simulink model "commpcccvs"  (R2023b)
settings: Solver=FixedStepDiscrete  StartTime=0.0  StopTime=360  RelTol=1e-3
PostLoadFcn:
  | %Default parameters
  | prmPcccVs.blkLength1 = 1024;
  | prmPcccVs.blkLength2 = 4096;
  | prmPcccVs.EbNo = 0.7;
  | prmPcccVs.numIter = 6;
  | 
  | % Derived parameter
  | prmPcccVs.maxBlkLength = max(prmPcccVs.blkLength1, prmPcccVs.blkLength2);
undefined symbols (not defined in the file or in its folder): gCRC24B, getTurboIOIndices
libraries: commsink2 x2, commdigbbndpm3 x2, commcrc2 x2, commrandsrc3 x2, dspsrcs4 x2, commcnvcod2 x2, commchan3 x1
Description:
  | Variable-sized Turbo Coding
  | 
  | Companion to the commpccc model, this model highlights Turbo coding with variable-sized signals in Simulink.
  | Using the 3GPP TS 36.212 v9.0 specifications for the Turbo encoder and decoder, the example
  | highlights the performance variations with different code block lengths.
  | 
  | The model can be configured to run with any two of the 188 code block sizes supported by the standard
  | and is set to evaluate the code block error performance over an AWGN channel.
settings Model: FPTRunName=Active  Creator=The MathWorks, Inc.  LastModifiedBy=yuvra
settings SolverCC: AlgebraicLoopSolver=TrustRegion
settings DataIOCC: LimitDataPoints=on  SaveFormat=Array  SaveOutput=off  SignalLogging=off  DSMLogging=off  SaveTime=off  ReturnWorkspaceOutputs=off
settings OptimizationCC: ReuseModelBlockBuffer=off  ExpressionDepthLimit=2147483647  RollThreshold=2  LifeSpan=inf  SimCompilerOptimization=on
settings DebuggingCC: UnderspecifiedInitializationDetection=Classic  MergeDetectMultiDrivingBlocksExec=none  SolverPrmCheckMsg=warning  FcnCallInpInsideContextMsg=warning  UnconnectedInputMsg=warning  UnconnectedOutputMsg=warning  UnconnectedLineMsg=warning  AllowSymbolicDim=off  StateNameClashWarn=warning  SFUnexpectedBacktrackingDiag=warning  SFNoUnconditionalDefaultTransitionDiag=warning  SFExecutionAtInitializationDiag=none  ArithmeticOperatorsInVariantConditions=warning
settings HardwareCC: ProdBitPerPointer=32  ProdBitPerSizeT=32  ProdBitPerPtrDiffT=32  ProdLargestAtomicFloat=None  ProdIntDivRoundTo=Undefined  ProdEndianess=Unspecified  ProdWordSize=32  ProdHWDeviceType=32-bit Generic
settings ModelReferenceCC: EnableRefExpFcnMdlSchedulingChecks=on  PropagateSignalLabelsOutOfModel=off
settings SFSimCC: SFSimEcho=off  SimCtrlC=off  SimIntegrity=off  SimUseLocalCustomCode=off  CustomCodeUndefinedFunction=UseInterfaceOnly
settings RTWCC: RTWUseLocalCustomCode=off  DLArmComputeVersion=19.05
settings CodeAppCC: StateflowObjectComments=on
settings GRTTargetCC: TargetLangStandard=C89/C90 (ANSI)  CombineOutputUpdateFcns=off  GRTInterface=on
settings ConfigComp: CovMetricSettings=dw  CovSaveCumulativeToWorkspaceVar=on  CovSaveSingleToWorkspaceVar=on  CovExternalEMLEnable=off  CovSFcnEnable=off

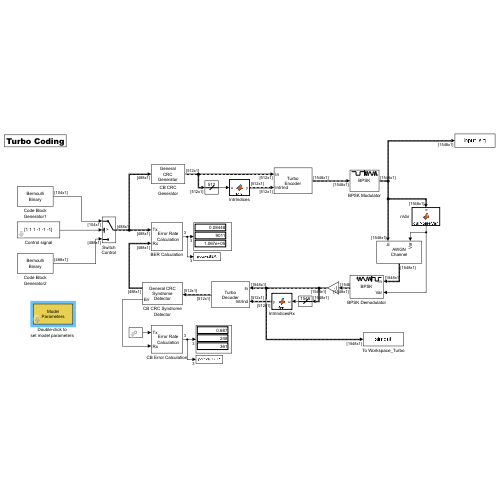
[thumbnail: Simulink's stored preview of the top-level diagram]
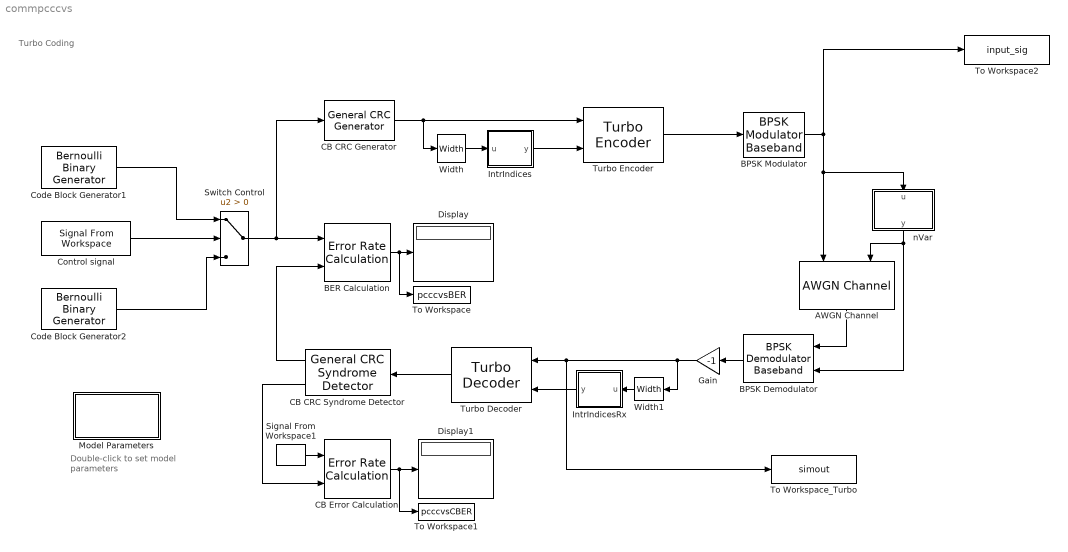
== system commpcccvs ==
  note: Turbo Coding
  note: Double-click to
      | set model parameters
  AWGN Channel : commchan3/AWGN Channel  LegacyMode=off  NoiseMethod=Variance  noiseMode=Variance from port  EbNo=10  EsNo=10  SNR=10  BitsPerSymbol=1  SignalPower=1  SamplesPerSymbol=1  SymbolPeriod=1  VarianceSource=Input port  Variance=1  RandomStream=mt19937ar with seed  Seed=98765  SimulateUsing=Code generation
  BER Calculation : commsink2/Error Rate Calculation  N=0  st_delay=0  cp_mode=Entire frame  subframe=[]  PMode=Port  WsName=ErrorVec1  RsMode2=off  stop=off  numErr=maxNumErrs  maxBits=maxNumBits
  BPSK Demodulator : commdigbbndpm3/BPSK Demodulator Baseband  DecType=Log-likelihood ratio  VarSource=Port  Variance=1  Ph=0  outDtype=Inherit via internal rule  derotateFactorWordLen=16  derotateFactorDataTypeStr=Inherit: Same word length as input  derotateFactorLastDataTypeStr=Inherit: Same word length as input
  BPSK Modulator : commdigbbndpm3/BPSK Modulator Baseband  Ph=0  outDtype=double  outWordLen=16  outUDDataType=sfix(16)  outFracLenMode=Best precision  outFracLen=15  outDataTypeStr=double  outLastDataTypeStr=double
  CB CRC Generator : commcrc2/General CRC Generator  genPoly=[1 1 zeros(1, 16) 1 1 0 0 0 1 1] % gCRC24B  iniStates=0  directMethod=off  reflectInputBytes=off  reflectChecksums=off  finalXOR=0  numChecksums=1
  CB CRC Syndrome Detector : commcrc2/General CRC Syndrome Detector  genPoly=[1 1 zeros(1, 16) 1 1 0 0 0 1 1] % gCRC24B  iniStates=0  directMethod=off  reflectInputBytes=off  reflectChecksums=off  finalXOR=0  numChecksums=1
  CB Error Calculation : commsink2/Error Rate Calculation  N=0  st_delay=0  cp_mode=Entire frame  subframe=[]  PMode=Port  WsName=ErrorVec1  RsMode2=off  stop=off  numErr=maxNumErrs  maxBits=maxNumBits
  Code Block Generator1 : commrandsrc3/Bernoulli Binary Generator  ProbabilityOfZero=0.5  SeedSource=Parameter  Seed=12345  SampleTime=1/(prmPcccVs.blkLength1-24)  SamplesPerFrame=prmPcccVs.blkLength1-24  OutputDataType=double  SimulateUsing=Interpreted execution
  Code Block Generator2 : commrandsrc3/Bernoulli Binary Generator  ProbabilityOfZero=0.5  SeedSource=Parameter  Seed=67890  SampleTime=1/(prmPcccVs.blkLength2-24)  SamplesPerFrame=prmPcccVs.blkLength2-24  OutputDataType=double  SimulateUsing=Interpreted execution
  Control signal : dspsrcs4/Signal From Workspace  X=[1 1 1 -1 -1 -1]  Ts=1  nsamps=1  OutputAfterFinalValue=Cyclic repetition  ignoreOrWarnInputAndFrameLengths=off  OutputFrames=on
  Display : Display
  Display1 : Display
  Gain : Gain  Gain=-1
  IntrIndices : MATLAB Function  TreatAsAtomicUnit=on
  IntrIndicesRx : MATLAB Function  TreatAsAtomicUnit=on
  Model Parameters : Subsystem  mask(Model Parameters){blkLength1=128, blkLength2=512, ebNo=0, numIter=6}
      mask prompts: blkLength1 "Code block length1 (bits):"; blkLength2 "Code block length2 (bits):"; ebNo "Eb/No (dB):"; numIter "Number of decoding iterations:"
      mask help: Specifies model parameters for a simulation run.
      mask init:
      | % Form the params structure
      | [p.blkLength1, p.blkLength2, p.EbNo, p.numIter] = deal(blkLength1, blkLength2, ebNo, numIter);
      | 
      | % Derived parameter
      | p.maxBlkLength = max(p.blkLength1, p.blkLength2);
      | 
      | % Assign variable to base workspace
      | assignin('base', 'prmPcccVs', p);
      mask Help: helpview(commdhelp);
      mask Display: disp('Model\nParameters');
  Signal From Workspace1 : dspsrcs4/Signal From Workspace  X=0  Ts=1  nsamps=1  OutputAfterFinalValue=Cyclic repetition  ignoreOrWarnInputAndFrameLengths=off  OutputFrames=on
  Switch Control : Switch  Criteria=u2 > Threshold  AllowDiffInputSizes=on  SaturateOnIntegerOverflow=off  InputSameDT=off
  To Workspace : ToWorkspace  VariableName=pcccvsBER  SampleTime=-1
      settings: MaxDataPoints=1
  To Workspace1 : ToWorkspace  VariableName=pcccvsCBER  SampleTime=-1
      settings: MaxDataPoints=1
  To Workspace2 : ToWorkspace  VariableName=input_sig  SaveFormat=Timeseries  SampleTime=-1
  To Workspace_Turbo : ToWorkspace  VariableName=simout  SaveFormat=Timeseries  SampleTime=-1
  Turbo Decoder : commcnvcod2/Turbo Decoder  TrellisStructure=poly2trellis( 4, [ 13, 15 ], 13 )  InterleaverIndicesSource=Input port  InterleaverIndices=(64:-1:1).'  InputIndicesSource=Auto  InputIndices=getTurboIOIndices( 64, 2, 3 )  Algorithm=True APP  NumScalingBits=3  NumIterations=prmPcccVs.numIter  SimulateUsing=Interpreted execution
  Turbo Encoder : commcnvcod2/Turbo Encoder  TrellisStructure=poly2trellis( 4, [ 13, 15 ], 13 )  InterleaverIndicesSource=Input port  InterleaverIndices=(64:-1:1).'  OutputIndicesSource=Auto  OutputIndices=getTurboIOIndices( 64, 2, 3 )  SimulateUsing=Interpreted execution
  Width : Width
  Width1 : Width
  nVar : MATLAB Function  TreatAsAtomicUnit=on
  wires:
  BER Calculation/1 -> Display/1, To Workspace/1
  BPSK Modulator/1 -> AWGN Channel/1, nVar/1(u), To Workspace2/1
  Turbo Encoder/1 -> BPSK Modulator/1
  IntrIndices/1(y) -> Turbo Encoder/2
  Control signal/1 -> Switch Control/2
  Code Block Generator2/1 -> Switch Control/3
  Switch Control/1 -> CB CRC Generator/1, BER Calculation/1
  Width1/1 -> IntrIndicesRx/1(u)
  IntrIndicesRx/1(y) -> Turbo Decoder/2
  nVar/1(y) -> AWGN Channel/2, BPSK Demodulator/2
  BPSK Demodulator/1 -> Gain/1
  AWGN Channel/1 -> BPSK Demodulator/1
  CB CRC Generator/1 -> Turbo Encoder/1, Width/1
  Turbo Decoder/1 -> CB CRC Syndrome Detector/1
  CB CRC Syndrome Detector/1 -> BER Calculation/2
  CB CRC Syndrome Detector/2 -> CB Error Calculation/2
  Signal From Workspace1/1 -> CB Error Calculation/1
  CB Error Calculation/1 -> Display1/1, To Workspace1/1
  Gain/1 -> To Workspace_Turbo/1, Turbo Decoder/1, Width1/1
  Width/1 -> IntrIndices/1(u)
  Code Block Generator1/1 -> Switch Control/1

== system commpcccvs/Model Parameters ==
  note: This subsystem is empty.
      | It is used for setting parameter values (in the mask).

== matlab function commpcccvs/nVar ==
  data: u input; y output; prmPcccVs parameter
function y = calNoiseVar(u, prmPcccVs)
%#codegen

inLen = size(u,1);
blkLen = (inLen/3)-4;
assert(blkLen>=40); assert(blkLen<=6144);

y = zeros(1, 1);

R = blkLen/inLen;
y = 1./(R*10^(0.1*prmPcccVs.EbNo));

== matlab function commpcccvs/IntrIndicesRx ==
  data: u input; y output size=[prmPcccVs.maxBlkLength 1]
function y = fcn(u)
%#codegen

x = (u/3)-4;
assert(x>=40); assert(x<=6144);
y = zeros(x, 1);

y = helperLTEIntrlvrIndices(x);

== matlab function commpcccvs/IntrIndices ==
  data: u input; y output size=[prmPcccVs.maxBlkLength 1]
function y = fcn(u)
%#codegen

assert(u>=40); assert(u<=6144);
y = zeros(u, 1);

y = helperLTEIntrlvrIndices(u);
